simulink model "secagem_de_graos_simulink"  (R2020a)
settings: Solver=VariableStepAuto  StartTime=0.0  StopTime=200  RelTol=1e-3
libraries: cstblocks x20
settings Model: Creator=Avell  LastModifiedBy=Avell

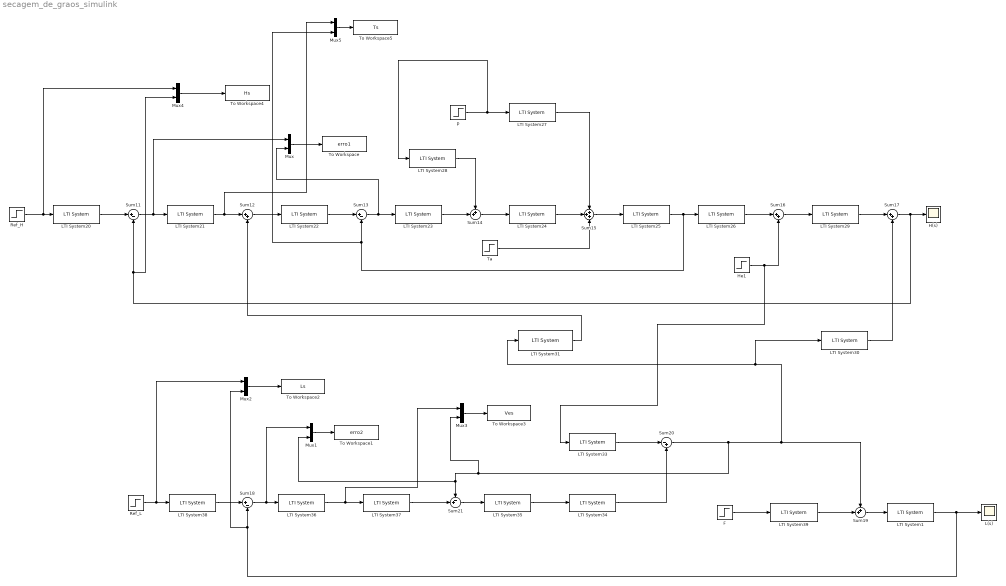
== system secagem_de_graos_simulink ==
  F : Step  Time=5  SampleTime=0
  H(s) : Scope
  He1 : Step  Time=20  SampleTime=0
  L(s) : Scope
  LTI System1 : cstblocks/LTI System  sys=G7  IC=[]
  LTI System20 : cstblocks/LTI System  sys=FCH  IC=[]
  LTI System21 : cstblocks/LTI System  sys=CH  IC=[]
  LTI System22 : cstblocks/LTI System  sys=FCT  IC=[]
  LTI System23 : cstblocks/LTI System  sys=CT  IC=[]
  LTI System24 : cstblocks/LTI System  sys=5  IC=[]
  LTI System25 : cstblocks/LTI System  sys=G1  IC=[]
  LTI System26 : cstblocks/LTI System  sys=5  IC=[]
  LTI System27 : cstblocks/LTI System  sys=2  IC=[]
  LTI System28 : cstblocks/LTI System  sys=Cffp  IC=[]
  LTI System29 : cstblocks/LTI System  sys=G2  IC=[]
  LTI System30 : cstblocks/LTI System  sys=G3  IC=[]
  LTI System31 : cstblocks/LTI System  sys=CffVe  IC=[]
  LTI System33 : cstblocks/LTI System  sys=G5  IC=[]
  LTI System34 : cstblocks/LTI System  sys=G6  IC=[]
  LTI System35 : cstblocks/LTI System  sys=CVe  IC=[]
  LTI System36 : cstblocks/LTI System  sys=CL  IC=[]
  LTI System37 : cstblocks/LTI System  sys=FCVe  IC=[]
  LTI System38 : cstblocks/LTI System  sys=FCL  IC=[]
  LTI System39 : cstblocks/LTI System  sys=G4  IC=[]
  Mux{,1..5} (6 alike) : Mux  Inputs=2
  Ref_H : Step  Time=50  SampleTime=0
  Ref_L : Step  Time=10  SampleTime=0
  Sum11 : Sum  Inputs=|+-
  Sum12 : Sum  Inputs=|++
  Sum13 : Sum  Inputs=|+-
  Sum14 : Sum  Inputs=++|
  Sum15 : Sum  Inputs=+++
  Sum16 : Sum  Inputs=|++
  Sum17 : Sum  Inputs=|++
  Sum18 : Sum  Inputs=|+-
  Sum19 : Sum  Inputs=++|
  Sum20 : Sum  Inputs=|-+
  Sum21 : Sum  Inputs=-+|
  Ta : Step  Time=7  SampleTime=0
  To Workspace : ToWorkspace  VariableName=erro1  SaveFormat=Structure With Time  SampleTime=-1
  To Workspace1 : ToWorkspace  VariableName=erro2  SaveFormat=Structure With Time  SampleTime=-1
  To Workspace2 : ToWorkspace  VariableName=Ls  SaveFormat=Structure With Time  SampleTime=-1
  To Workspace3 : ToWorkspace  VariableName=Ves  SaveFormat=Structure With Time  SampleTime=-1
  To Workspace4 : ToWorkspace  VariableName=Hs  SaveFormat=Structure With Time  SampleTime=-1
  To Workspace5 : ToWorkspace  VariableName=Ts  SaveFormat=Structure With Time  SampleTime=-1
  p : Step  Time=10  SampleTime=0
  wires:
  Ref_H/1 -> Mux4/1, LTI System20/1
  LTI System20/1 -> Sum11/1
  Sum11/1 -> Mux/1, LTI System21/1
  LTI System21/1 -> Mux5/1, Sum12/1
  Sum12/1 -> LTI System22/1
  LTI System22/1 -> Sum13/1
  Sum13/1 -> Mux/2, LTI System23/1
  LTI System23/1 -> Sum14/2
  Sum14/1 -> LTI System24/1
  LTI System24/1 -> Sum15/2
  Sum15/1 -> LTI System25/1
  LTI System25/1 -> Mux5/2, Sum13/2, LTI System26/1
  p/1 -> LTI System27/1, LTI System28/1
  LTI System26/1 -> Sum16/1
  Sum16/1 -> LTI System29/1
  LTI System29/1 -> Sum17/1
  Sum17/1 -> Mux4/2, Sum11/2, H(s)/1
  Sum20/1 -> Sum19/1, LTI System30/1, LTI System31/1, Mux3/2, Mux1/2, Sum21/1
  He1/1 -> LTI System33/1, Sum16/2
  Ta/1 -> Sum15/3
  LTI System27/1 -> Sum15/1
  LTI System28/1 -> Sum14/1
  LTI System31/1 -> Sum12/2
  LTI System30/1 -> Sum17/2
  LTI System37/1 -> Sum21/2
  LTI System36/1 -> Mux3/1, LTI System37/1
  Ref_L/1 -> Mux2/1, LTI System38/1
  Sum18/1 -> Mux1/1, LTI System36/1
  LTI System35/1 -> LTI System34/1
  Sum21/1 -> LTI System35/1
  LTI System38/1 -> Sum18/1
  LTI System33/1 -> Sum20/1
  LTI System34/1 -> Sum20/2
  Sum19/1 -> LTI System1/1
  LTI System39/1 -> Sum19/2
  F/1 -> LTI System39/1
  Mux/1 -> To Workspace/1
  Mux1/1 -> To Workspace1/1
  Mux2/1 -> To Workspace2/1
  LTI System1/1 -> Mux2/2, Sum18/2, L(s)/1
  Mux3/1 -> To Workspace3/1
  Mux4/1 -> To Workspace4/1
  Mux5/1 -> To Workspace5/1
